simulink model "simscape_thermofluids_full"  (R2024b)
settings: Solver=VariableStepAuto  StartTime=0.0  StopTime=stopTime  FixedStep=timestep
values from neighbouring files (symbols this model uses):
  AC_tank_weight = AC_wall_thickness*AC_tank_surface_area*steel_density*2    [design_details.m]
  Ambient_temp = 300    [design_details.m]
  hose_length = 20    [design_details.m]
  Initial_temp = 300    [design_details.m]
  mass_per_length_supply = steel_density*wall_thickness*(supply_pipe_inner_area + supply_pipe_outer_area)    [design_details.m]
  supply_pipe_inner_diameter = 0.05    [design_details.m]
  wall_thickness = 2/1000    (= 0.002)    [design_details.m]
undefined symbols (not defined in the file or in its folder): AC_Bypass_SOV_POS, AC_Engine_SOV_POS, AC_Return_SOV_POS, AC_Supply_SOV_POS, GH2_PROP_VALVE_POS, GS_GH2_SOV_POS, GS_RETURN_PROP_POS, GS_Return_SOV_POS, GS_Supply_SOV_POS, LH2_PROP_VALVE_POS, mass_per_length_engine_feed, P_BYPASS, P_COUPLING_AC, P_COUPLING_AC_RETURN, P_COUPLINGS_GS, P_ENGINE_FEED, P_GH2_SUPPLY_GS, P_HOSE_GS, P_HOSE_RETURN_GS, P_PUMP_GS, P_SOV_RETURN_GS, P_TANK_AC, P_TANK_GS, P_VALVE_GS, T_BYPASS, T_COUPLING_AC, T_COUPLING_AC_RETURN, T_COUPLINGS_GS, T_ENGINE_FEED, T_GH2_SUPPLY_GS, T_HOSE_GS, T_HOSE_RETURN_GS, T_PUMP_GS, T_SOV_RETURN_GS, T_TANK_AC, T_TANK_GS, T_VALVE_GS
libraries: fl_lib x75, nesl_utility x62, SimscapeFluids_lib x14
(part 1 of 2)
settings Model: Creator=MW  LastModifiedBy=MW
settings SolverCC: SolverResetMethod=Robust

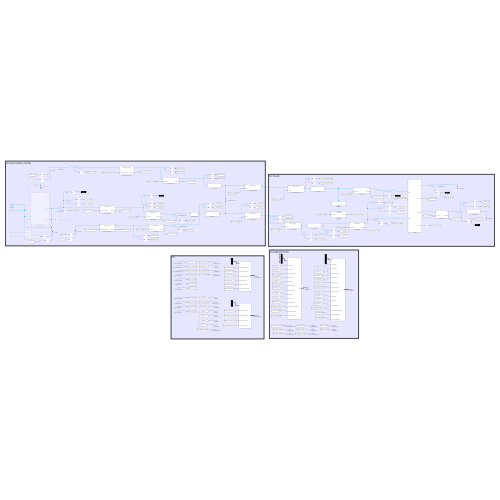
[thumbnail: Simulink's stored preview of the top-level diagram]
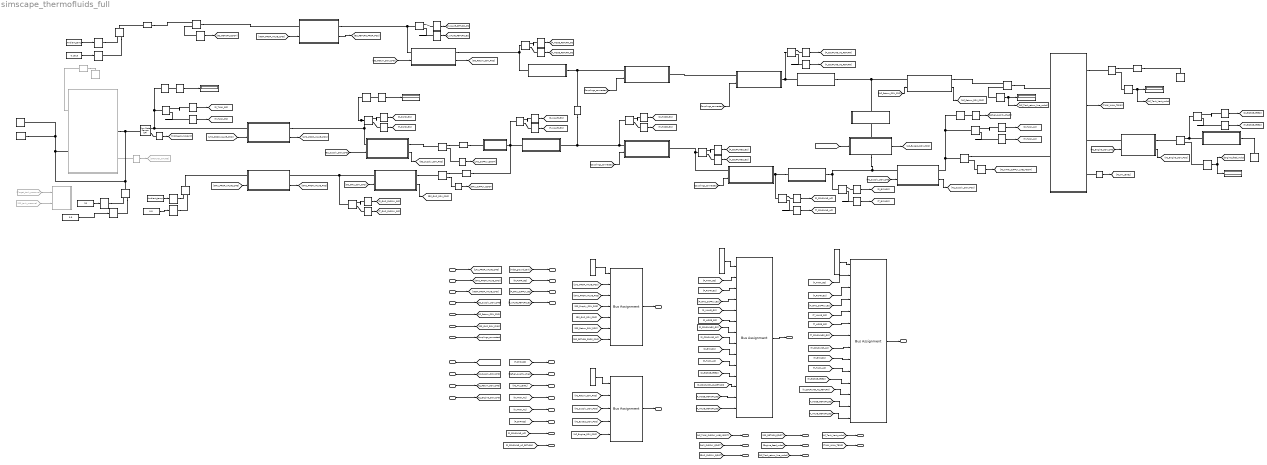
== system simscape_thermofluids_full ==
  note: Ground station fluids
  note: I/O
  note: AC fluids
  note: DIAGNOSTICS
  LH2_PROP_VALVE_CMD : Inport  OutDataTypeStr=double
  GH2_PROP_VALVE_CMD : Inport  Port=2
  VENT_PROP_VALVE_CMD : Inport  Port=3
  GS_Supply_SOV_CMD : Inport  Port=4  OutDataTypeStr=boolean
  GS_Return_SOV_CMD : Inport  Port=5  OutDataTypeStr=boolean
  GS_GH2_SOV_CMD : Inport  Port=6  OutDataTypeStr=boolean
  Couplings_connected : Inport  Port=7  OutDataTypeStr=boolean
  AC_Bypass_SOV_CMD : Inport  Port=8  OutDataTypeStr=boolean
  AC_Supply_SOV_CMD : Inport  Port=9  OutDataTypeStr=boolean
  AC_Return_SOV_CMD : Inport  Port=10  OutDataTypeStr=boolean
  AC_Engine_SOV_CMD : Inport  Port=11  OutDataTypeStr=boolean
  AC bypass check valve : SimscapeFluids_lib/Two-Phase Fluid/Valves & Orifices/Directional Control Valves/Check Valve (2P)  liquid_valve_parameterization=fluids.two_phase_fluid.valves_orifices.enum.LiquidPressureValveParameterization.LinearArea  opening_pressure_spec=fluids.two_phase_fluid.valves_orifices.enum.PressureControlSpec.PressureDifferential  p_crack_differential=1 bar  p_crack_gauge=0.1 MPa  p_max_differential=1.2 bar  p_max_gauge=0.2 MPa  mdot_nominal_max=0.1 kg/s  delta_p_nominal_max=0.001 MPa  valve_area_max=return_valve_orifice_area m^2  p_diff_TLU=[0.2 : 0.2 : 1.2] MPa  p_gauge_TLU=[0.2 : 0.2 : 1.2] MPa  valve_area_TLU=[1e-10, 2e-06, 4e-06, 6e-06, 8e-06, 1e-05] m^2  energy_spec=foundation.enum.energy_spec.temperature  p_inlet=0.101325 MPa  T_inlet=293.15 K  x_inlet=0  alpha_inlet=0  h_inlet=400 kJ/kg  u_inlet=400 kJ/kg  Cd=0.8  pressure_recovery=false  leakage_fraction=1e-9  smoothing_factor=0.01  B_lam=0.999  tau_x=0.1 s  area=return_pipe_inner_area m^2  vapor_valve_parameterization=fluids.two_phase_fluid.valves_orifices.enum.VaporOrificeParameterization.Cv  opening_characteristic=fluids.two_phase_fluid.valves_orifices.enum.OpeningCharacteristics.Linear  Cv_max=4  p_diff_Cv_TLU=0.2 : 0.2 : 1.2 MPa  p_gauge_Cv_TLU=0.2 : 0.2 : 1.2 MPa  Cv_TLU=[1e-06, .8, 1.6, 2.4, 3.2, 4]  xT_Cv=0.7  Kv_max=3.6  p_diff_Kv_TLU=0.2 : 0.2 : 1.2 MPa  p_gauge_Kv_TLU=0.2 : 0.2 : 1.2 MPa  Kv_TLU=[1e-06, .72, 1.44, 2.16, 2.88, 3.6]  xT_Kv=0.7  orifice_area_max=1e-4 m^2  p_diff_orifice_area_TLU=0.2 : 0.2 : 1.2 MPa  p_gauge_orifice_area_TLU=0.2 : 0.2 : 1.2 MPa  orifice_area_TLU=[1e-10, 2e-05, 4e-05, 6e-05, 8e-05, .0001] m^2
      settings: InternalSimscapePortConfiguration="{\"Bottom\":[],\"Left\":[{\"id\":\"A\",\"label\":\"A\",\"type\":\"foundation.two_phase_fluid.two_phase_fluid\"}],\"Right\":[{\"id\":\"B\",\"label\":\"B\",\"type\":\"foundation.two_phase_fluid.two_phase_fluid\"}],\"Top\":[]}"
  AC bypass pipe : Subsystem
      settings: PortSchema="{\"entries\":[{\"content\":{\"sides\":[{\"content\":{},\"type\":\"ConnectorPlacement.EquallySpacedRectSide\",\"uuid\":\"349fca2d-ac0c-44ed-9349-b644fbb08439\"},{\"content\":{\"side\":\"RIGHT\"},\"type\":\"ConnectorPlacement.EquallySpacedRectSide\",\"uuid\":\"6cc07318-8be0-4b72-ac83-45de534072f6\"},{\"content\":{\"connectorIds\":[\"LConn1\"],\"side\":\"TOP\"},\"type\":\"ConnectorPlacement.EquallySpacedRectSide\",\"uuid\":\"b4ae9877-c592-4d5d-8aa9-db7f627bda4a\"},{\"content\":{\"connectorIds\":[\"RConn1\"],\"side\":\"BOTTOM\"},\"type\":\"ConnectorPlacement.EquallySpacedRectSide\",\"uuid\":\"fa6d3200-a15a-4c5e-bc85-f306dce7b3ce\"}]},\"type\":\"ConnectorPlacement.EquallySpacedConnector\",\"uuid\":\"04c81fd1-333a-4337-ad58-fb71ace63568\"}],\"packageUris\":[\"http://schema.mathworks.com/mf0/Connector/R2020b\"],\"version\":\"1.0\"}"
  AC engine_feed_pipe : Subsystem
  AC return line pipe : Subsystem
  AC supply line pipe : Subsystem
  AC tank : Subsystem
      settings: PortSchema="{\"entries\":[{\"content\":{\"sides\":[{\"content\":{\"connectorIds\":[\"LConn1\",\"LConn2\"]},\"type\":\"ConnectorPlacement.EquallySpacedRectSide\",\"uuid\":\"18fbfd65-7892-4f33-871e-6daf68ba144c\"},{\"content\":{\"connectorIds\":[\"RConn1\",\"Out1\",\"RConn2\",\"RConn3\"],\"side\":\"RIGHT\"},\"type\":\"ConnectorPlacement.EquallySpacedRectSide\",\"uuid\":\"09c519c2-126c-4ac0-b88b-b8c0f8bd496e\"},{\"content\":{\"side\":\"TOP\"},\"type\":\"ConnectorPlacement.EquallySpacedRectSide\",\"uuid\":\"0da44e65-d94a-4bbc-a863-04d0cc4fadcc\"}]},\"type\":\"ConnectorPlacement.EquallySpacedConnector\",\"uuid\":\"f3f4eab3-fa1f-4341-9602-c44ab5467c31\"}],\"packageUris\":[\"http://schema.mathworks.com/mf0/Connector/R2020b\"],\"version\":\"1.0\"}"
  AC tank safety valve : SimscapeFluids_lib/Two-Phase Fluid/Valves & Orifices/Directional Control Valves/Check Valve (2P)  liquid_valve_parameterization=fluids.two_phase_fluid.valves_orifices.enum.LiquidPressureValveParameterization.LinearArea  opening_pressure_spec=fluids.two_phase_fluid.valves_orifices.enum.PressureControlSpec.PressureDifferential  p_crack_differential=5.5 bar  p_crack_gauge=0.1 MPa  p_max_differential=5.9 bar  p_max_gauge=0.2 MPa  mdot_nominal_max=0.1 kg/s  delta_p_nominal_max=0.001 MPa  valve_area_max=return_valve_orifice_area m^2  p_diff_TLU=[0.2 : 0.2 : 1.2] MPa  p_gauge_TLU=[0.2 : 0.2 : 1.2] MPa  valve_area_TLU=[1e-10, 2e-06, 4e-06, 6e-06, 8e-06, 1e-05] m^2  energy_spec=foundation.enum.energy_spec.temperature  p_inlet=0.101325 MPa  T_inlet=293.15 K  x_inlet=0  alpha_inlet=0  h_inlet=400 kJ/kg  u_inlet=400 kJ/kg  Cd=0.64  pressure_recovery=false  leakage_fraction=1e-9  smoothing_factor=0.01  B_lam=0.999  tau_x=0.1 s  area=return_pipe_inner_area m^2  vapor_valve_parameterization=fluids.two_phase_fluid.valves_orifices.enum.VaporOrificeParameterization.Cv  opening_characteristic=fluids.two_phase_fluid.valves_orifices.enum.OpeningCharacteristics.Linear  Cv_max=4  p_diff_Cv_TLU=0.2 : 0.2 : 1.2 MPa  p_gauge_Cv_TLU=0.2 : 0.2 : 1.2 MPa  Cv_TLU=[1e-06, .8, 1.6, 2.4, 3.2, 4]  xT_Cv=0.7  Kv_max=3.6  p_diff_Kv_TLU=0.2 : 0.2 : 1.2 MPa  p_gauge_Kv_TLU=0.2 : 0.2 : 1.2 MPa  Kv_TLU=[1e-06, .72, 1.44, 2.16, 2.88, 3.6]  xT_Kv=0.7  orifice_area_max=1e-4 m^2  p_diff_orifice_area_TLU=0.2 : 0.2 : 1.2 MPa  p_gauge_orifice_area_TLU=0.2 : 0.2 : 1.2 MPa  orifice_area_TLU=[1e-10, 2e-05, 4e-05, 6e-05, 8e-05, .0001] m^2
      settings: InternalSimscapePortConfiguration="{\"Bottom\":[],\"Left\":[{\"id\":\"A\",\"label\":\"A\",\"type\":\"foundation.two_phase_fluid.two_phase_fluid\"}],\"Right\":[{\"id\":\"B\",\"label\":\"B\",\"type\":\"foundation.two_phase_fluid.two_phase_fluid\"}],\"Top\":[]}"
  AC_Bypass_SOV : Subsystem  ReferencedSubsystem=liquid_supply_SOV
      settings: PortSchema="{\"entries\":[{\"content\":{\"sides\":[{\"content\":{\"connectorIds\":[\"In1\"]},\"type\":\"ConnectorPlacement.EquallySpacedRectSide\",\"uuid\":\"7761104f-7ea1-4b82-8256-1f0a81ecff04\"},{\"content\":{\"connectorIds\":[\"Out1\"],\"side\":\"RIGHT\"},\"type\":\"ConnectorPlacement.EquallySpacedRectSide\",\"uuid\":\"77ad54b1-fc7d-49b0-961f-dd624ba54eaa\"},{\"content\":{\"connectorIds\":[\"RConn1\"],\"side\":\"TOP\"},\"type\":\"ConnectorPlacement.EquallySpacedRectSide\",\"uuid\":\"3eb2c4da-9d99-4a14-9c12-4cb71cddfd05\"},{\"content\":{\"connectorIds\":[\"LConn1\"],\"side\":\"BOTTOM\"},\"type\":\"ConnectorPlacement.EquallySpacedRectSide\",\"uuid\":\"cc93d467-c3c5-4ce4-93ce-594b4fdbf767\"}]},\"type\":\"ConnectorPlacement.EquallySpacedConnector\",\"uuid\":\"a385487e-9e14-4b1e-bbba-76ef306222d1\"}],\"packageUris\":[\"http://schema.mathworks.com/mf0/Connector/R2020b\"],\"version\":\"1.0\"}"
  AC_Engine_SOV : Subsystem
      settings: PortSchema="{\"entries\":[{\"content\":{\"sides\":[{\"content\":{\"connectorIds\":[\"LConn1\",\"In1\"]},\"type\":\"ConnectorPlacement.EquallySpacedRectSide\",\"uuid\":\"8de00a24-9637-44f9-b77e-5b0008e83c26\"},{\"content\":{\"connectorIds\":[\"RConn1\",\"Out1\"],\"side\":\"RIGHT\"},\"type\":\"ConnectorPlacement.EquallySpacedRectSide\",\"uuid\":\"a538d446-b2a2-4ee6-8065-c38203dba177\"},{\"content\":{\"side\":\"TOP\"},\"type\":\"ConnectorPlacement.EquallySpacedRectSide\",\"uuid\":\"7c3a0b8e-131f-419e-9dd3-9151f58d9c4d\"}]},\"type\":\"ConnectorPlacement.EquallySpacedConnector\",\"uuid\":\"82546791-8f2d-494c-94b0-dfe79e322a77\"}],\"packageUris\":[\"http://schema.mathworks.com/mf0/Connector/R2020b\"],\"version\":\"1.0\"}"
  AC_Return_Coupling : Subsystem  ReferencedSubsystem=Return_coupling
      settings: PortSchema="{\"entries\":[{\"content\":{\"sides\":[{\"content\":{\"connectorIds\":[\"LConn1\",\"In1\"]},\"type\":\"ConnectorPlacement.EquallySpacedRectSide\",\"uuid\":\"1377ff57-d661-4db4-88bf-068b5be5647d\"},{\"content\":{\"connectorIds\":[\"RConn1\"],\"side\":\"RIGHT\"},\"type\":\"ConnectorPlacement.EquallySpacedRectSide\",\"uuid\":\"b2bd98a1-a4a4-4b83-ae68-33d4546d1bd4\"},{\"content\":{\"side\":\"TOP\"},\"type\":\"ConnectorPlacement.EquallySpacedRectSide\",\"uuid\":\"bd2d13e7-0124-4459-acb6-2626b7f191a3\"}]},\"type\":\"ConnectorPlacement.EquallySpacedConnector\",\"uuid\":\"1a0dd594-d6c0-4a46-87d8-aae9dae4eba9\"}],\"packageUris\":[\"http://schema.mathworks.com/mf0/Connector/R2020b\"],\"version\":\"1.0\"}"
  AC_Return_SOV : Subsystem
      settings: PortSchema="{\"entries\":[{\"content\":{\"sides\":[{\"content\":{\"connectorIds\":[\"LConn1\",\"In1\"]},\"type\":\"ConnectorPlacement.EquallySpacedRectSide\",\"uuid\":\"1377ff57-d661-4db4-88bf-068b5be5647d\"},{\"content\":{\"connectorIds\":[\"RConn1\",\"Out1\"],\"side\":\"RIGHT\"},\"type\":\"ConnectorPlacement.EquallySpacedRectSide\",\"uuid\":\"b2bd98a1-a4a4-4b83-ae68-33d4546d1bd4\"},{\"content\":{\"side\":\"TOP\"},\"type\":\"ConnectorPlacement.EquallySpacedRectSide\",\"uuid\":\"bd2d13e7-0124-4459-acb6-2626b7f191a3\"},{\"content\":{\"side\":\"BOTTOM\"},\"type\":\"ConnectorPlacement.EquallySpacedRectSide\",\"uuid\":\"65261db1-7dc3-4c3c-a5c1-ee0ef291cfbc\"}]},\"type\":\"ConnectorPlacement.EquallySpacedConnector\",\"uuid\":\"1a0dd594-d6c0-4a46-87d8-aae9dae4eba9\"}],\"packageUris\":[\"http://schema.mathworks.com/mf0/Connector/R2020b\"],\"version\":\"1.0\"}"
  AC_Supply_Coupling : Subsystem  ReferencedSubsystem=Supply_coupling
      settings: PortSchema="{\"entries\":[{\"content\":{\"sides\":[{\"content\":{\"connectorIds\":[\"LConn1\",\"In1\"]},\"type\":\"ConnectorPlacement.EquallySpacedRectSide\",\"uuid\":\"1377ff57-d661-4db4-88bf-068b5be5647d\"},{\"content\":{\"connectorIds\":[\"RConn1\"],\"side\":\"RIGHT\"},\"type\":\"ConnectorPlacement.EquallySpacedRectSide\",\"uuid\":\"b2bd98a1-a4a4-4b83-ae68-33d4546d1bd4\"},{\"content\":{\"side\":\"TOP\"},\"type\":\"ConnectorPlacement.EquallySpacedRectSide\",\"uuid\":\"bd2d13e7-0124-4459-acb6-2626b7f191a3\"}]},\"type\":\"ConnectorPlacement.EquallySpacedConnector\",\"uuid\":\"1a0dd594-d6c0-4a46-87d8-aae9dae4eba9\"}],\"packageUris\":[\"http://schema.mathworks.com/mf0/Connector/R2020b\"],\"version\":\"1.0\"}"
  AC_Supply_SOV : Subsystem  ReferencedSubsystem=liquid_supply_SOV
      settings: PortSchema="{\"entries\":[{\"content\":{\"sides\":[{\"content\":{\"connectorIds\":[\"LConn1\",\"In1\"]},\"type\":\"ConnectorPlacement.EquallySpacedRectSide\",\"uuid\":\"7761104f-7ea1-4b82-8256-1f0a81ecff04\"},{\"content\":{\"connectorIds\":[\"RConn1\",\"Out1\"],\"side\":\"RIGHT\"},\"type\":\"ConnectorPlacement.EquallySpacedRectSide\",\"uuid\":\"77ad54b1-fc7d-49b0-961f-dd624ba54eaa\"},{\"content\":{\"side\":\"TOP\"},\"type\":\"ConnectorPlacement.EquallySpacedRectSide\",\"uuid\":\"3eb2c4da-9d99-4a14-9c12-4cb71cddfd05\"}]},\"type\":\"ConnectorPlacement.EquallySpacedConnector\",\"uuid\":\"a385487e-9e14-4b1e-bbba-76ef306222d1\"}],\"packageUris\":[\"http://schema.mathworks.com/mf0/Connector/R2020b\"],\"version\":\"1.0\"}"
  Atmosphere : fl_lib/Two-Phase Fluid/Elements/Reservoir (2P)  Commented=on  pressure_spec=foundation.enum.ReservoirPressureSpec2P.Specified  reservoir_pressure=0.101325 MPa  reservoir_condensing_temperature=373.15 K  reservoir_evaporating_temperature=373.15 K  energy_spec=foundation.enum.ReservoirEnergySpec2P.Temperature  reservoir_temperature=Ambient_temp K  reservoir_quality=0.5  reservoir_void_fraction=0.5  reservoir_enthalpy=1500 kJ/kg  reservoir_internal_energy=1500 kJ/kg  reservoir_subcooling=5 deltaK  reservoir_superheating=5 deltaK  area_A=0.01 m^2
  Atmosphere2 : fl_lib/Two-Phase Fluid/Elements/Reservoir (2P)  pressure_spec=foundation.enum.ReservoirPressureSpec2P.Specified  reservoir_pressure=0.101325 MPa  reservoir_condensing_temperature=373.15 K  reservoir_evaporating_temperature=373.15 K  energy_spec=foundation.enum.ReservoirEnergySpec2P.Temperature  reservoir_temperature=293.15 K  reservoir_quality=0.5  reservoir_void_fraction=0.5  reservoir_enthalpy=1500 kJ/kg  reservoir_internal_energy=1500 kJ/kg  reservoir_subcooling=5 deltaK  reservoir_superheating=5 deltaK  area_A=0.02 m^2
  Atmosphere3 : fl_lib/Two-Phase Fluid/Elements/Reservoir (2P)  pressure_spec=foundation.enum.ReservoirPressureSpec2P.Specified  reservoir_pressure=0.101325 MPa  reservoir_condensing_temperature=373.15 K  reservoir_evaporating_temperature=373.15 K  energy_spec=foundation.enum.ReservoirEnergySpec2P.Temperature  reservoir_temperature=Ambient_temp K  reservoir_quality=0.5  reservoir_void_fraction=0.5  reservoir_enthalpy=1500 kJ/kg  reservoir_internal_energy=1500 kJ/kg  reservoir_subcooling=5 deltaK  reservoir_superheating=5 deltaK  area_A=engine_feed_pipe_inner_area m^2
  Bus Assignment : BusAssignment  AssignedSignals=P_TANK_GS,P_PUMP_GS,P_GH2_SUPPLY_GS,P_VALVE_GS,P_HOSE_GS,P_COUPLINGS_GS,P_COUPLING_AC,P_BYPASS,P_TANK_AC,P_ENGINE_FEED,P_COUPLING_AC_RETURN,P_HOSE_RETURN_GS,P_SOV_RETURN_GS
  Bus Assignment1 : BusAssignment  AssignedSignals=T_TANK_GS,T_PUMP_GS,T_GH2_SUPPLY_GS,T_VALVE_GS,T_HOSE_GS,T_COUPLINGS_GS,T_COUPLING_AC,T_BYPASS,T_TANK_AC,T_ENGINE_FEED,T_COUPLING_AC_RETURN,T_HOSE_RETURN_GS,T_SOV_RETURN_GS
  Bus Assignment2 : BusAssignment  AssignedSignals=LH2_PROP_VALVE_POS,GH2_PROP_VALVE_POS,GS_Supply_SOV_POS,GS_GH2_SOV_POS,GS_Return_SOV_POS,GS_RETURN_PROP_POS
  Bus Assignment3 : BusAssignment  AssignedSignals=AC_Return_SOV_POS,AC_Supply_SOV_POS,AC_Bypass_SOV_POS,AC_Engine_SOV_POS
  Bus Creator : BusCreator  Inputs=13  OutDataTypeStr=Bus: P_DIAGNOSTIC  NonVirtualBus=on
      settings: InheritFromInputs=off
  Bus Creator1 : BusCreator  Inputs=13  OutDataTypeStr=Bus: T_DIAGNOSTIC  NonVirtualBus=on
      settings: InheritFromInputs=off
  Bus Creator2 : BusCreator  Inputs=6  OutDataTypeStr=Bus: GS_VALVE_FEEDBACK  NonVirtualBus=on
      settings: InheritFromInputs=off
  Bus Creator3 : BusCreator  Inputs=4  OutDataTypeStr=Bus: AC_VALVE_FEEDBACK  NonVirtualBus=on
      settings: InheritFromInputs=off
  Constant : Constant  Value=Ambient_temp
  Constant1 : Constant  Value=20
  Constant2 : Constant  Value=Ambient_temp
  Constant4 : Constant  Value=0.5
  Constant5 : Constant  Value=0.1013
  Constant6 : Constant  Value=0.5
  Display{,1..4} (5 alike) : Display
  Flow Rate Sensor (2P) : fl_lib/Two-Phase Fluid/Sensors/Flow Rate Sensor (2P)  mass_flow_measure=false  volumetric_flow_measure=true  energy_flow_measure=false
      settings: InternalSimscapePortConfiguration="{\"Bottom\":[],\"Left\":[{\"id\":\"A\",\"label\":\"A\",\"type\":\"foundation.two_phase_fluid.two_phase_fluid\"}],\"Right\":[{\"id\":\"B\",\"label\":\"B\",\"type\":\"foundation.two_phase_fluid.two_phase_fluid\"},{\"id\":\"V\",\"label\":\"V\",\"type\":\"output\"}],\"Top\":[]}"
  Flow Rate Sensor (2P)1 : fl_lib/Two-Phase Fluid/Sensors/Flow Rate Sensor (2P)  mass_flow_measure=false  volumetric_flow_measure=true  energy_flow_measure=false
      settings: InternalSimscapePortConfiguration="{\"Bottom\":[],\"Left\":[{\"id\":\"A\",\"label\":\"A\",\"type\":\"foundation.two_phase_fluid.two_phase_fluid\"}],\"Right\":[{\"id\":\"B\",\"label\":\"B\",\"type\":\"foundation.two_phase_fluid.two_phase_fluid\"},{\"id\":\"V\",\"label\":\"V\",\"type\":\"output\"}],\"Top\":[]}"
  Flow Rate Sensor (2P){2..3,5..6} (4 alike) : fl_lib/Two-Phase Fluid/Sensors/Flow Rate Sensor (2P)  mass_flow_measure=true  volumetric_flow_measure=false  energy_flow_measure=false
      settings: InternalSimscapePortConfiguration="{\"Bottom\":[],\"Left\":[{\"id\":\"A\",\"label\":\"A\",\"type\":\"foundation.two_phase_fluid.two_phase_fluid\"}],\"Right\":[{\"id\":\"B\",\"label\":\"B\",\"type\":\"foundation.two_phase_fluid.two_phase_fluid\"},{\"id\":\"M\",\"label\":\"M\",\"type\":\"output\"}],\"Top\":[]}"
  Flow Rate Sensor (2P)4 : fl_lib/Two-Phase Fluid/Sensors/Flow Rate Sensor (2P)  mass_flow_measure=false  volumetric_flow_measure=true  energy_flow_measure=false
      settings: InternalSimscapePortConfiguration="{\"Bottom\":[],\"Left\":[{\"id\":\"A\",\"label\":\"A\",\"type\":\"foundation.two_phase_fluid.two_phase_fluid\"}],\"Right\":[{\"id\":\"B\",\"label\":\"B\",\"type\":\"foundation.two_phase_fluid.two_phase_fluid\"},{\"id\":\"V\",\"label\":\"V\",\"type\":\"output\"}],\"Top\":[]}"
  Flow rate sensor : fl_lib/Two-Phase Fluid/Sensors/Flow Rate Sensor (2P)  mass_flow_measure=true  volumetric_flow_measure=false  energy_flow_measure=false
      settings: InternalSimscapePortConfiguration="{\"Bottom\":[],\"Left\":[{\"id\":\"A\",\"label\":\"A\",\"type\":\"foundation.two_phase_fluid.two_phase_fluid\"}],\"Right\":[{\"id\":\"B\",\"label\":\"B\",\"type\":\"foundation.two_phase_fluid.two_phase_fluid\"},{\"id\":\"M\",\"label\":\"M\",\"type\":\"output\"}],\"Top\":[]}"
  From : From  Commented=on  GotoTag=Target_tank_pressure
  From14 : From  Commented=on  GotoTag=GS_tank_pressure
  GH2 Proportional valve : Subsystem  ReferencedSubsystem=Gas_prop_valve
      settings: PortSchema="{\"entries\":[{\"content\":{\"sides\":[{\"content\":{\"connectorIds\":[\"LConn1\",\"In1\"]},\"type\":\"ConnectorPlacement.EquallySpacedRectSide\",\"uuid\":\"7761104f-7ea1-4b82-8256-1f0a81ecff04\"},{\"content\":{\"connectorIds\":[\"LConn2\",\"Out1\"],\"side\":\"RIGHT\"},\"type\":\"ConnectorPlacement.EquallySpacedRectSide\",\"uuid\":\"77ad54b1-fc7d-49b0-961f-dd624ba54eaa\"},{\"content\":{\"side\":\"TOP\"},\"type\":\"ConnectorPlacement.EquallySpacedRectSide\",\"uuid\":\"3eb2c4da-9d99-4a14-9c12-4cb71cddfd05\"},{\"content\":{\"side\":\"BOTTOM\"},\"type\":\"ConnectorPlacement.EquallySpacedRectSide\",\"uuid\":\"e49cc93b-8c4a-4262-8b13-a5abe2820965\"}]},\"type\":\"ConnectorPlacement.EquallySpacedConnector\",\"uuid\":\"a385487e-9e14-4b1e-bbba-76ef306222d1\"}],\"packageUris\":[\"http://schema.mathworks.com/mf0/Connector/R2020b\"],\"version\":\"1.0\"}"
  GH2 source : fl_lib/Two-Phase Fluid/Elements/Controlled Reservoir (2P)  pressure_spec=foundation.enum.ControlledReservoirPressureSpec2P.Specified  energy_spec=foundation.enum.ControlledReservoirEnergySpec2P.VaporTemperature  area_A=supply_valve_orifice_area m^2  pressure_limit_spec=foundation.enum.PressureLimitSpec2P.Warn
      settings: InternalSimscapePortConfiguration="{\"Bottom\":[],\"Left\":[{\"id\":\"A\",\"label\":\"A\",\"type\":\"foundation.two_phase_fluid.two_phase_fluid\"}],\"Right\":[{\"id\":\"T\",\"label\":\"T\",\"type\":\"input\"},{\"id\":\"P\",\"label\":\"P\",\"type\":\"input\"}],\"Top\":[]}"
  GH2 supply check valve : SimscapeFluids_lib/Two-Phase Fluid/Valves & Orifices/Directional Control Valves/Check Valve (2P)  liquid_valve_parameterization=fluids.two_phase_fluid.valves_orifices.enum.LiquidPressureValveParameterization.LinearArea  opening_pressure_spec=fluids.two_phase_fluid.valves_orifices.enum.PressureControlSpec.PressureDifferential  p_crack_differential=0.01 bar  p_crack_gauge=0.1 MPa  p_max_differential=0.03 bar  p_max_gauge=0.2 MPa  mdot_nominal_max=0.1 kg/s  delta_p_nominal_max=0.001 MPa  valve_area_max=supply_valve_orifice_area m^2  p_diff_TLU=[0.2 : 0.2 : 1.2] MPa  p_gauge_TLU=[0.2 : 0.2 : 1.2] MPa  valve_area_TLU=[1e-10, 2e-06, 4e-06, 6e-06, 8e-06, 1e-05] m^2  energy_spec=foundation.enum.energy_spec.temperature  p_inlet=0.101325 MPa  T_inlet=293.15 K  x_inlet=0  alpha_inlet=0  h_inlet=400 kJ/kg  u_inlet=400 kJ/kg  Cd=0.8  pressure_recovery=false  leakage_fraction=1e-9  smoothing_factor=0.01  B_lam=0.999  tau_x=0.1 s  area=supply_pipe_inner_area m^2  vapor_valve_parameterization=fluids.two_phase_fluid.valves_orifices.enum.VaporOrificeParameterization.Cv  opening_characteristic=fluids.two_phase_fluid.valves_orifices.enum.OpeningCharacteristics.Linear  Cv_max=4  p_diff_Cv_TLU=0.2 : 0.2 : 1.2 MPa  p_gauge_Cv_TLU=0.2 : 0.2 : 1.2 MPa  Cv_TLU=[1e-06, .8, 1.6, 2.4, 3.2, 4]  xT_Cv=0.7  Kv_max=3.6  p_diff_Kv_TLU=0.2 : 0.2 : 1.2 MPa  p_gauge_Kv_TLU=0.2 : 0.2 : 1.2 MPa  Kv_TLU=[1e-06, .72, 1.44, 2.16, 2.88, 3.6]  xT_Kv=0.7  orifice_area_max=1e-4 m^2  p_diff_orifice_area_TLU=0.2 : 0.2 : 1.2 MPa  p_gauge_orifice_area_TLU=0.2 : 0.2 : 1.2 MPa  orifice_area_TLU=[1e-10, 2e-05, 4e-05, 6e-05, 8e-05, .0001] m^2
      settings: InternalSimscapePortConfiguration="{\"Bottom\":[],\"Left\":[{\"id\":\"A\",\"label\":\"A\",\"type\":\"foundation.two_phase_fluid.two_phase_fluid\"}],\"Right\":[{\"id\":\"B\",\"label\":\"B\",\"type\":\"foundation.two_phase_fluid.two_phase_fluid\"}],\"Top\":[]}"
  GH2 vent : fl_lib/Two-Phase Fluid/Elements/Controlled Reservoir (2P)  pressure_spec=foundation.enum.ControlledReservoirPressureSpec2P.Specified  energy_spec=foundation.enum.ControlledReservoirEnergySpec2P.VaporTemperature  area_A=supply_valve_orifice_area m^2  pressure_limit_spec=foundation.enum.PressureLimitSpec2P.Warn
      settings: InternalSimscapePortConfiguration="{\"Bottom\":[],\"Left\":[{\"id\":\"A\",\"label\":\"A\",\"type\":\"foundation.two_phase_fluid.two_phase_fluid\"}],\"Right\":[{\"id\":\"T\",\"label\":\"T\",\"type\":\"input\"},{\"id\":\"P\",\"label\":\"P\",\"type\":\"input\"}],\"Top\":[]}"
  GS supply line pipe : Subsystem
  GS tank pressure controller : Subsystem  Commented=on
  GS_GH2_SOV : Subsystem  ReferencedSubsystem=liquid_supply_SOV
      settings: PortSchema="{\"entries\":[{\"content\":{\"sides\":[{\"content\":{\"connectorIds\":[\"LConn1\",\"In1\"]},\"type\":\"ConnectorPlacement.EquallySpacedRectSide\",\"uuid\":\"7761104f-7ea1-4b82-8256-1f0a81ecff04\"},{\"content\":{\"connectorIds\":[\"RConn1\",\"Out1\"],\"side\":\"RIGHT\"},\"type\":\"ConnectorPlacement.EquallySpacedRectSide\",\"uuid\":\"77ad54b1-fc7d-49b0-961f-dd624ba54eaa\"},{\"content\":{\"side\":\"TOP\"},\"type\":\"ConnectorPlacement.EquallySpacedRectSide\",\"uuid\":\"3eb2c4da-9d99-4a14-9c12-4cb71cddfd05\"}]},\"type\":\"ConnectorPlacement.EquallySpacedConnector\",\"uuid\":\"a385487e-9e14-4b1e-bbba-76ef306222d1\"}],\"packageUris\":[\"http://schema.mathworks.com/mf0/Connector/R2020b\"],\"version\":\"1.0\"}"
  GS_Return_Coupling : Subsystem  ReferencedSubsystem=Return_coupling
      settings: PortSchema="{\"entries\":[{\"content\":{\"sides\":[{\"content\":{\"connectorIds\":[\"LConn1\",\"In1\"]},\"type\":\"ConnectorPlacement.EquallySpacedRectSide\",\"uuid\":\"1377ff57-d661-4db4-88bf-068b5be5647d\"},{\"content\":{\"connectorIds\":[\"RConn1\"],\"side\":\"RIGHT\"},\"type\":\"ConnectorPlacement.EquallySpacedRectSide\",\"uuid\":\"b2bd98a1-a4a4-4b83-ae68-33d4546d1bd4\"},{\"content\":{\"side\":\"TOP\"},\"type\":\"ConnectorPlacement.EquallySpacedRectSide\",\"uuid\":\"bd2d13e7-0124-4459-acb6-2626b7f191a3\"}]},\"type\":\"ConnectorPlacement.EquallySpacedConnector\",\"uuid\":\"1a0dd594-d6c0-4a46-87d8-aae9dae4eba9\"}],\"packageUris\":[\"http://schema.mathworks.com/mf0/Connector/R2020b\"],\"version\":\"1.0\"}"
  GS_Return_SOV : Subsystem
      settings: PortSchema="{\"entries\":[{\"content\":{\"sides\":[{\"content\":{\"connectorIds\":[\"LConn1\",\"In1\"]},\"type\":\"ConnectorPlacement.EquallySpacedRectSide\",\"uuid\":\"1377ff57-d661-4db4-88bf-068b5be5647d\"},{\"content\":{\"connectorIds\":[\"RConn1\",\"Out1\"],\"side\":\"RIGHT\"},\"type\":\"ConnectorPlacement.EquallySpacedRectSide\",\"uuid\":\"b2bd98a1-a4a4-4b83-ae68-33d4546d1bd4\"},{\"content\":{\"side\":\"TOP\"},\"type\":\"ConnectorPlacement.EquallySpacedRectSide\",\"uuid\":\"bd2d13e7-0124-4459-acb6-2626b7f191a3\"}]},\"type\":\"ConnectorPlacement.EquallySpacedConnector\",\"uuid\":\"1a0dd594-d6c0-4a46-87d8-aae9dae4eba9\"}],\"packageUris\":[\"http://schema.mathworks.com/mf0/Connector/R2020b\"],\"version\":\"1.0\"}"
  GS_Supply_Coupling : Subsystem  ReferencedSubsystem=Supply_coupling
      settings: PortSchema="{\"entries\":[{\"content\":{\"sides\":[{\"content\":{\"connectorIds\":[\"LConn1\",\"In1\"]},\"type\":\"ConnectorPlacement.EquallySpacedRectSide\",\"uuid\":\"1377ff57-d661-4db4-88bf-068b5be5647d\"},{\"content\":{\"connectorIds\":[\"RConn1\"],\"side\":\"RIGHT\"},\"type\":\"ConnectorPlacement.EquallySpacedRectSide\",\"uuid\":\"b2bd98a1-a4a4-4b83-ae68-33d4546d1bd4\"},{\"content\":{\"side\":\"TOP\"},\"type\":\"ConnectorPlacement.EquallySpacedRectSide\",\"uuid\":\"bd2d13e7-0124-4459-acb6-2626b7f191a3\"}]},\"type\":\"ConnectorPlacement.EquallySpacedConnector\",\"uuid\":\"1a0dd594-d6c0-4a46-87d8-aae9dae4eba9\"}],\"packageUris\":[\"http://schema.mathworks.com/mf0/Connector/R2020b\"],\"version\":\"1.0\"}"
  GS_Supply_SOV : Subsystem  ReferencedSubsystem=liquid_supply_SOV
      settings: PortSchema="{\"entries\":[{\"content\":{\"sides\":[{\"content\":{\"connectorIds\":[\"LConn1\",\"In1\"]},\"type\":\"ConnectorPlacement.EquallySpacedRectSide\",\"uuid\":\"7761104f-7ea1-4b82-8256-1f0a81ecff04\"},{\"content\":{\"connectorIds\":[\"RConn1\",\"Out1\"],\"side\":\"RIGHT\"},\"type\":\"ConnectorPlacement.EquallySpacedRectSide\",\"uuid\":\"77ad54b1-fc7d-49b0-961f-dd624ba54eaa\"},{\"content\":{\"side\":\"TOP\"},\"type\":\"ConnectorPlacement.EquallySpacedRectSide\",\"uuid\":\"3eb2c4da-9d99-4a14-9c12-4cb71cddfd05\"}]},\"type\":\"ConnectorPlacement.EquallySpacedConnector\",\"uuid\":\"a385487e-9e14-4b1e-bbba-76ef306222d1\"}],\"packageUris\":[\"http://schema.mathworks.com/mf0/Connector/R2020b\"],\"version\":\"1.0\"}"
  Goto1 : Goto  Commented=on  GotoTag=GROUND_GAUGE
  Ground station tank : Subsystem  Commented=on
  H2 2 phase : fl_lib/Two-Phase Fluid/Utilities/Two-Phase Fluid Properties (2P)  u_min=H2Tables.u_min kJ/kg  u_max=H2Tables.u_max kJ/kg  p_TLU=H2Tables.p MPa  p_crit=H2Tables.p_crit MPa  critical_region=foundation.enum.critical_region.clip  p_crit_fraction=0.12  p_atm=0.101325 MPa  properties_range_check=simscape.enum.assert.action.error  q_rev=0.01 Pa  unorm_liq=H2Tables.liquid.unorm  v_liq=H2Tables.liquid.v m^3/kg  s_liq=H2Tables.liquid.s kJ/(kg*K)  T_liq=H2Tables.liquid.T K  nu_liq=H2Tables.liquid.nu mm^2/s  k_liq=H2Tables.liquid.k W/(m*K)  Pr_liq=H2Tables.liquid.Pr  u_sat_liq=H2Tables.liquid.u_sat kJ/kg  unorm_vap=H2Tables.vapor.unorm  v_vap=H2Tables.vapor.v m^3/kg  s_vap=H2Tables.vapor.s kJ/(kg*K)  T_vap=H2Tables.vapor.T K  nu_vap=H2Tables.vapor.nu mm^2/s  k_vap=H2Tables.vapor.k W/(m*K)  Pr_vap=H2Tables.vapor.Pr  u_sat_vap=H2Tables.vapor.u_sat kJ/kg
      settings: InternalSimscapePortConfiguration="{\"Bottom\":[],\"Left\":[],\"Right\":[{\"id\":\"A\",\"label\":\"\",\"type\":\"foundation.two_phase_fluid.two_phase_fluid\"}],\"Top\":[]}"
  LH2 Proportional valve : Subsystem  ReferencedSubsystem=LH2_prop_valve
      settings: PortSchema="{\"entries\":[{\"content\":{\"sides\":[{\"content\":{\"connectorIds\":[\"LConn1\",\"In1\"]},\"type\":\"ConnectorPlacement.EquallySpacedRectSide\",\"uuid\":\"feebead4-63a3-41be-b6af-c9093fc48b74\"},{\"content\":{\"connectorIds\":[\"LConn2\",\"Out1\"],\"side\":\"RIGHT\"},\"type\":\"ConnectorPlacement.EquallySpacedRectSide\",\"uuid\":\"7fa0aa45-6202-479f-80c3-49b7dbf56766\"},{\"content\":{\"side\":\"TOP\"},\"type\":\"ConnectorPlacement.EquallySpacedRectSide\",\"uuid\":\"fffd3c2c-2b50-47ce-80c6-79193e21f29e\"},{\"content\":{\"side\":\"BOTTOM\"},\"type\":\"ConnectorPlacement.EquallySpacedRectSide\",\"uuid\":\"957ddecd-60b1-4a90-a8a1-75fcc228f543\"}]},\"type\":\"ConnectorPlacement.EquallySpacedConnector\",\"uuid\":\"476b1e20-77c8-4bf2-b4c4-536305065543\"}],\"packageUris\":[\"http://schema.mathworks.com/mf0/Connector/R2020b\"],\"version\":\"1.0\"}"
  LH2 source : fl_lib/Two-Phase Fluid/Elements/Controlled Reservoir (2P)  pressure_spec=foundation.enum.ControlledReservoirPressureSpec2P.Specified  energy_spec=foundation.enum.ControlledReservoirEnergySpec2P.LiquidTemperature  area_A=0.1 m^2  pressure_limit_spec=foundation.enum.PressureLimitSpec2P.Limit
      settings: InternalSimscapePortConfiguration="{\"Bottom\":[],\"Left\":[{\"id\":\"A\",\"label\":\"A\",\"type\":\"foundation.two_phase_fluid.two_phase_fluid\"}],\"Right\":[{\"id\":\"T\",\"label\":\"T\",\"type\":\"input\"},{\"id\":\"P\",\"label\":\"P\",\"type\":\"input\"}],\"Top\":[]}"
  LH2 supply check valve : SimscapeFluids_lib/Two-Phase Fluid/Valves & Orifices/Directional Control Valves/Check Valve (2P)  liquid_valve_parameterization=fluids.two_phase_fluid.valves_orifices.enum.LiquidPressureValveParameterization.LinearArea  opening_pressure_spec=fluids.two_phase_fluid.valves_orifices.enum.PressureControlSpec.PressureDifferential  p_crack_differential=0.01 bar  p_crack_gauge=0.1 MPa  p_max_differential=0.03 bar  p_max_gauge=0.2 MPa  mdot_nominal_max=0.1 kg/s  delta_p_nominal_max=0.001 MPa  valve_area_max=supply_valve_orifice_area m^2  p_diff_TLU=[0.2 : 0.2 : 1.2] MPa  p_gauge_TLU=[0.2 : 0.2 : 1.2] MPa  valve_area_TLU=[1e-10, 2e-06, 4e-06, 6e-06, 8e-06, 1e-05] m^2  energy_spec=foundation.enum.energy_spec.temperature  p_inlet=0.101325 MPa  T_inlet=293.15 K  x_inlet=0  alpha_inlet=0  h_inlet=400 kJ/kg  u_inlet=400 kJ/kg  Cd=0.8  pressure_recovery=false  leakage_fraction=1e-9  smoothing_factor=0.01  B_lam=0.999  tau_x=0.1 s  area=supply_pipe_inner_area m^2  vapor_valve_parameterization=fluids.two_phase_fluid.valves_orifices.enum.VaporOrificeParameterization.Cv  opening_characteristic=fluids.two_phase_fluid.valves_orifices.enum.OpeningCharacteristics.Linear  Cv_max=4  p_diff_Cv_TLU=0.2 : 0.2 : 1.2 MPa  p_gauge_Cv_TLU=0.2 : 0.2 : 1.2 MPa  Cv_TLU=[1e-06, .8, 1.6, 2.4, 3.2, 4]  xT_Cv=0.7  Kv_max=3.6  p_diff_Kv_TLU=0.2 : 0.2 : 1.2 MPa  p_gauge_Kv_TLU=0.2 : 0.2 : 1.2 MPa  Kv_TLU=[1e-06, .72, 1.44, 2.16, 2.88, 3.6]  xT_Kv=0.7  orifice_area_max=1e-4 m^2  p_diff_orifice_area_TLU=0.2 : 0.2 : 1.2 MPa  p_gauge_orifice_area_TLU=0.2 : 0.2 : 1.2 MPa  orifice_area_TLU=[1e-10, 2e-05, 4e-05, 6e-05, 8e-05, .0001] m^2
      settings: InternalSimscapePortConfiguration="{\"Bottom\":[],\"Left\":[{\"id\":\"A\",\"label\":\"A\",\"type\":\"foundation.two_phase_fluid.two_phase_fluid\"}],\"Right\":[{\"id\":\"B\",\"label\":\"B\",\"type\":\"foundation.two_phase_fluid.two_phase_fluid\"}],\"Top\":[]}"
  PS-Simulink Converter{,1,3..38} (38 alike) : nesl_utility/PS-Simulink Converter  PhysicalDomain=network_engine_domain  SubClassName=ps_output  LeftPortType=input  RightPortType=output  PseudoPeriodic=off  Frequencies=[]  VectorFormat=inherit  Unit=inherit  AffineConversion=off
  PS-Simulink Converter2 : nesl_utility/PS-Simulink Converter  Commented=on  PhysicalDomain=network_engine_domain  SubClassName=ps_output  LeftPortType=input  RightPortType=output  PseudoPeriodic=off  Frequencies=[]  VectorFormat=inherit  Unit=inherit  AffineConversion=off
  Pressure, Temperature & Internal Energy Sensor (2P){,1..12} (13 alike) : fl_lib/Two-Phase Fluid/Sensors/Pressure, Temperature & Internal Energy Sensor (2P)  reference=foundation.enum.MeasurementReference.absolute  pressure=true  pressure_spec=foundation.enum.PressureMeasementSpec.Absolute  temperature=true  internal_energy=false
      settings: InternalSimscapePortConfiguration="{\"Bottom\":[{\"id\":\"T\",\"label\":\"T\",\"type\":\"output\"}],\"Left\":[{\"id\":\"A\",\"label\":\"A\",\"type\":\"foundation.two_phase_fluid.two_phase_fluid\"}],\"Right\":[{\"id\":\"Pa\",\"label\":\"Pa\",\"type\":\"output\"}],\"Top\":[]}"
  Return gas proportional valve : Subsystem  ReferencedSubsystem=Return_gas_prop_valve
      settings: PortSchema="{\"entries\":[{\"content\":{\"sides\":[{\"content\":{\"connectorIds\":[\"LConn2\",\"In1\"]},\"type\":\"ConnectorPlacement.EquallySpacedRectSide\",\"uuid\":\"7b60590b-4a7b-465d-b616-9ce36d4c9bd1\"},{\"content\":{\"connectorIds\":[\"LConn1\",\"Out1\"],\"side\":\"RIGHT\"},\"type\":\"ConnectorPlacement.EquallySpacedRectSide\",\"uuid\":\"021f4d26-2a2b-40fc-b211-2c38ffe0620d\"},{\"content\":{\"side\":\"TOP\"},\"type\":\"ConnectorPlacement.EquallySpacedRectSide\",\"uuid\":\"273f71b8-2e8c-4f2f-b50f-0419d15b1792\"}]},\"type\":\"ConnectorPlacement.EquallySpacedConnector\",\"uuid\":\"b42a82ba-0baa-43b5-8ff8-ec1372f42070\"}],\"packageUris\":[\"http://schema.mathworks.com/mf0/Connector/R2020b\"],\"version\":\"1.0\"}"
  Return line hose : Subsystem
  Safety valve : SimscapeFluids_lib/Two-Phase Fluid/Valves & Orifices/Directional Control Valves/Check Valve (2P)  Commented=on  liquid_valve_parameterization=fluids.two_phase_fluid.valves_orifices.enum.LiquidPressureValveParameterization.LinearArea  opening_pressure_spec=fluids.two_phase_fluid.valves_orifices.enum.PressureControlSpec.PressureDifferential  p_crack_differential=6 bar  p_crack_gauge=0.1 MPa  p_max_differential=7 bar  p_max_gauge=0.2 MPa  mdot_nominal_max=0.1 kg/s  delta_p_nominal_max=0.001 MPa  valve_area_max=1e-2 m^2  p_diff_TLU=[0.2 : 0.2 : 1.2] MPa  p_gauge_TLU=[0.2 : 0.2 : 1.2] MPa  valve_area_TLU=[1e-10, 2e-06, 4e-06, 6e-06, 8e-06, 1e-05] m^2  energy_spec=foundation.enum.energy_spec.temperature  p_inlet=0.101325 MPa  T_inlet=293.15 K  x_inlet=0  alpha_inlet=0  h_inlet=400 kJ/kg  u_inlet=400 kJ/kg  Cd=0.64  pressure_recovery=false  leakage_fraction=1e-9  smoothing_factor=0.01  B_lam=0.999  tau_x=0.1 s  area=0.02 m^2  vapor_valve_parameterization=fluids.two_phase_fluid.valves_orifices.enum.VaporOrificeParameterization.Cv  opening_characteristic=fluids.two_phase_fluid.valves_orifices.enum.OpeningCharacteristics.Linear  Cv_max=4  p_diff_Cv_TLU=0.2 : 0.2 : 1.2 MPa  p_gauge_Cv_TLU=0.2 : 0.2 : 1.2 MPa  Cv_TLU=[1e-06, .8, 1.6, 2.4, 3.2, 4]  xT_Cv=0.7  Kv_max=3.6  p_diff_Kv_TLU=0.2 : 0.2 : 1.2 MPa  p_gauge_Kv_TLU=0.2 : 0.2 : 1.2 MPa  Kv_TLU=[1e-06, .72, 1.44, 2.16, 2.88, 3.6]  xT_Kv=0.7  orifice_area_max=1e-4 m^2  p_diff_orifice_area_TLU=0.2 : 0.2 : 1.2 MPa  p_gauge_orifice_area_TLU=0.2 : 0.2 : 1.2 MPa  orifice_area_TLU=[1e-10, 2e-05, 4e-05, 6e-05, 8e-05, .0001] m^2
      settings: InternalSimscapePortConfiguration="{\"Bottom\":[],\"Left\":[{\"id\":\"A\",\"label\":\"A\",\"type\":\"foundation.two_phase_fluid.two_phase_fluid\"}],\"Right\":[{\"id\":\"B\",\"label\":\"B\",\"type\":\"foundation.two_phase_fluid.two_phase_fluid\"}],\"Top\":[]}"
  Simulink-PS Converter{,1..5} (6 alike) : nesl_utility/Simulink-PS Converter  PhysicalDomain=network_engine_domain  SubClassName=ps_input  LeftPortType=input  RightPortType=output  PseudoPeriodic=off  Frequencies=[]  NoiseDistribution=none  NoiseParameters=[]  Unit=1  AffineConversion=off  FilteringAndDerivatives=provide  SimscapeFilterOrder=1  InputFilterTimeConstant=0.001  UdotUserProvided=0
  Solver Configuration2 : nesl_utility/Solver Configuration  PhysicalDomain=network_engine_domain  SubClassName=solver  LeftPortType=input  RightPortType=generic  Tones=[]  Harmonics=[]  SimulateNoise=off  Profile=off  UseLocalSampling=off  EnableSwitchedLinearOptims=on  FrequencyDomain=off  UseCCode=off  RelTol=0.001  AbsTol=0.001  MinStep=1e-09  ToWorkspace=off  RevertToSquareIcSolve=off  NumHomotopyIterations=100  PhasorMode=off  PhasorModeNumHarmonics=1  ConsistencySolver=NEWTON_XTOL_AFTER_FTOL  IndexReductionMethod=DerivativeReplacement  DoDC=off  ResidualTolerance=1e-09  ConsistencyTolSource=GLOBAL  ConsistencyAbsTol=0.001  ConsistencyRelTol=0.001  ConsistencyTolFactor=1e-7  UseLocalSolver=off  LocalSolverChoice=NE_TRAPEZOIDAL_ADVANCER  ResolveIndetEquations=on  FunctionEvalNumThread=1  LocalSolverSampleTime=1e-3  DoFixedCost=off  MaxNonlinIter=3  MaxModeIter=2  ComputeImpulses=off  ImpulseIterations=2  LinearAlgebra=auto  LinearAlgebraNumThread=0  EquationFormulation=NE_TIME_EF  DelaysMemoryBudget=1024  AutomaticFiltering=on  FilteringTimeConstant=0.001  PartitionStorageMethod=AS_NEEDED  PartitionMemoryBudget=1024  PartitionMethod=ROBUST  MultibodyUseLocalSolver=off  MultibodyLocalSolverChoice=ODE1  MultibodyLocalSolverSampleTime=0.001
  Vapor Quality Sensor (2P) : fl_lib/Two-Phase Fluid/Sensors/Vapor Quality Sensor (2P)  vapor_fraction_spec=foundation.enum.vapor_fraction_spec.quality
      settings: InternalSimscapePortConfiguration="{\"Bottom\":[],\"Left\":[{\"id\":\"A\",\"label\":\"A\",\"type\":\"foundation.two_phase_fluid.two_phase_fluid\"}],\"Right\":[{\"id\":\"X\",\"label\":\"X\",\"type\":\"output\"}],\"Top\":[]}"
  Vapor Quality Sensor (2P)1 : fl_lib/Two-Phase Fluid/Sensors/Vapor Quality Sensor (2P)  vapor_fraction_spec=foundation.enum.vapor_fraction_spec.quality
      settings: InternalSimscapePortConfiguration="{\"Bottom\":[],\"Left\":[{\"id\":\"A\",\"label\":\"A\",\"type\":\"foundation.two_phase_fluid.two_phase_fluid\"}],\"Right\":[{\"id\":\"X\",\"label\":\"X\",\"type\":\"output\"}],\"Top\":[]}"
  Vapor Quality Sensor (2P)2 : fl_lib/Two-Phase Fluid/Sensors/Vapor Quality Sensor (2P)  vapor_fraction_spec=foundation.enum.vapor_fraction_spec.quality
      settings: InternalSimscapePortConfiguration="{\"Bottom\":[],\"Left\":[{\"id\":\"A\",\"label\":\"A\",\"type\":\"foundation.two_phase_fluid.two_phase_fluid\"}],\"Right\":[{\"id\":\"X\",\"label\":\"X\",\"type\":\"output\"}],\"Top\":[]}"
  Vent check valve : SimscapeFluids_lib/Two-Phase Fluid/Valves & Orifices/Directional Control Valves/Check Valve (2P)  liquid_valve_parameterization=fluids.two_phase_fluid.valves_orifices.enum.LiquidPressureValveParameterization.LinearArea  opening_pressure_spec=fluids.two_phase_fluid.valves_orifices.enum.PressureControlSpec.PressureDifferential  p_crack_differential=0.01 bar  p_crack_gauge=0.1 MPa  p_max_differential=0.03 bar  p_max_gauge=0.2 MPa  mdot_nominal_max=0.1 kg/s  delta_p_nominal_max=0.001 MPa  valve_area_max=return_valve_orifice_area m^2  p_diff_TLU=[0.2 : 0.2 : 1.2] MPa  p_gauge_TLU=[0.2 : 0.2 : 1.2] MPa  valve_area_TLU=[1e-10, 2e-06, 4e-06, 6e-06, 8e-06, 1e-05] m^2  energy_spec=foundation.enum.energy_spec.temperature  p_inlet=0.101325 MPa  T_inlet=293.15 K  x_inlet=0  alpha_inlet=0  h_inlet=400 kJ/kg  u_inlet=400 kJ/kg  Cd=0.8  pressure_recovery=false  leakage_fraction=1e-9  smoothing_factor=0.01  B_lam=0.999  tau_x=0.1 s  area=return_pipe_inner_area m^2  vapor_valve_parameterization=fluids.two_phase_fluid.valves_orifices.enum.VaporOrificeParameterization.Cv  opening_characteristic=fluids.two_phase_fluid.valves_orifices.enum.OpeningCharacteristics.Linear  Cv_max=4  p_diff_Cv_TLU=0.2 : 0.2 : 1.2 MPa  p_gauge_Cv_TLU=0.2 : 0.2 : 1.2 MPa  Cv_TLU=[1e-06, .8, 1.6, 2.4, 3.2, 4]  xT_Cv=0.7  Kv_max=3.6  p_diff_Kv_TLU=0.2 : 0.2 : 1.2 MPa  p_gauge_Kv_TLU=0.2 : 0.2 : 1.2 MPa  Kv_TLU=[1e-06, .72, 1.44, 2.16, 2.88, 3.6]  xT_Kv=0.7  orifice_area_max=1e-4 m^2  p_diff_orifice_area_TLU=0.2 : 0.2 : 1.2 MPa  p_gauge_orifice_area_TLU=0.2 : 0.2 : 1.2 MPa  orifice_area_TLU=[1e-10, 2e-05, 4e-05, 6e-05, 8e-05, .0001] m^2
      settings: InternalSimscapePortConfiguration="{\"Bottom\":[],\"Left\":[{\"id\":\"A\",\"label\":\"A\",\"type\":\"foundation.two_phase_fluid.two_phase_fluid\"}],\"Right\":[{\"id\":\"B\",\"label\":\"B\",\"type\":\"foundation.two_phase_fluid.two_phase_fluid\"}],\"Top\":[]}"
  supply line hose : Subsystem
  mdot_ground_tank : Outport
  P_PUMP_GS : Outport  Port=2
  P_GH2_SUPPLY_GS : Outport  Port=3
  P_VALVE_RETURN_GS : Outport  Port=4
  T_BYPASS : Outport  Port=5
  Refuel_quality_check : Outport  Port=6
  AC_TK_LEVEL : Outport  Port=7
  P_TANK_AC : Outport  Port=8
  T_TANK_AC : Outport  Port=9
  P_BYPASS : Outport  Port=10
  P_COUPLING_AC : Outport  Port=11
  P_COUPLING_AC_RETURN : Outport  Port=12
  P_DIAGNOSTIC : Outport  Port=13  OutDataTypeStr=Bus: P_DIAGNOSTIC
  T_DIAGNOSTIC : Outport  Port=14  OutDataTypeStr=Bus: T_DIAGNOSTIC
  AC_TANK_SUPPLY_LINE_MDOT : Outport  Port=15
  LH2_SUPPLY_QDOT : Outport  Port=16
  GH2_SUPPLY_QDOT : Outport  Port=17
  GS_RETURN_QDOT : Outport  Port=18
  Engine_feed_mdot : Outport  Port=19
  AC_Tank_return_line_mdot : Outport  Port=20
  AC_Tank_Vent_mdot : Outport  Port=21
  Tank wall temp : Outport  Port=22
  GS_VALVE_FEEDBACK : Outport  Port=23  OutDataTypeStr=Bus: GS_VALVE_FEEDBACK
  AC_VALVE_FEEDBACK : Outport  Port=24  OutDataTypeStr=Bus: AC_VALVE_FEEDBACK
  wires:
  PS-Simulink Converter/1 -> [T_BYPASS]
  From/1 -> GS tank pressure controller/1(Target pressure)
  [Couplings_connected] -> GS_Return_Coupling/1
  Couplings_connected/1 -> [Couplings_connected]
  PS-Simulink Converter2/1 -> Goto1/1
  [mdot_ground_tank] -> mdot_ground_tank/1
  [Couplings_connected] -> AC_Supply_Coupling/1
  PS-Simulink Converter3/1 -> [AC_TK_LEVEL]
  PS-Simulink Converter4/1 -> [Refuel_quality_check]
  [Couplings_connected] -> AC_Return_Coupling/1
  [GS_Supply_SOV_CMD] -> GS_Supply_SOV/1
  [AC_Return_SOV_CMD] -> AC_Return_SOV/1(Valve_command)
  PS-Simulink Converter1/1 -> [mdot_ground_tank]
  [AC_Supply_SOV_CMD] -> AC_Supply_SOV/1
  [AC_Bypass_SOV_CMD] -> AC_Bypass_SOV/1
  From14/1 -> GS tank pressure controller/2(Tank pressure)
  [AC_Engine_SOV_CMD] -> AC_Engine_SOV/1(Valve_command)
  [GS_Return_SOV_CMD] -> GS_Return_SOV/1(Valve_command)
  [Couplings_connected] -> GS_Supply_Coupling/1
  GS_Supply_SOV_CMD/1 -> [GS_Supply_SOV_CMD]
  GS_Return_SOV_CMD/1 -> [GS_Return_SOV_CMD]
  AC_Supply_SOV_CMD/1 -> [AC_Supply_SOV_CMD]
  AC_Return_SOV_CMD/1 -> [AC_Return_SOV_CMD]
  AC_Bypass_SOV_CMD/1 -> [AC_Bypass_SOV_CMD]
  AC_Engine_SOV_CMD/1 -> [AC_Engine_SOV_CMD]
  [T_BYPASS] -> T_BYPASS/1
  [Refuel_quality_check] -> Refuel_quality_check/1
  [AC_TK_LEVEL] -> AC_TK_LEVEL/1
  PS-Simulink Converter5/1 -> [T_TANK_AC]
  PS-Simulink Converter6/1 -> [P_TANK_AC]
  [P_TANK_AC] -> P_TANK_AC/1
  [T_TANK_AC] -> T_TANK_AC/1
  PS-Simulink Converter8/1 -> [P_TANK_GS]
  PS-Simulink Converter7/1 -> [T_TANK_GS]
  PS-Simulink Converter9/1 -> [P_BYPASS]
  [P_BYPASS] -> P_BYPASS/1
  PS-Simulink Converter14/1 -> [T_VALVE_GS]
  PS-Simulink Converter15/1 -> [P_VALVE_GS]
  PS-Simulink Converter17/1 -> [P_HOSE_GS]
  PS-Simulink Converter16/1 -> [T_HOSE_GS]
  [P_TANK_GS] -> Bus Assignment/2
  Bus Assignment/1 -> P_DIAGNOSTIC/1
  [T_TANK_GS] -> Bus Assignment1/2
  Bus Assignment1/1 -> T_DIAGNOSTIC/1
  PS-Simulink Converter18/1 -> [T_COUPLINGS_GS]
  PS-Simulink Converter19/1 -> [P_COUPLINGS_GS]
  [GS_GH2_SOV_CMD] -> GS_GH2_SOV/1
  GS_GH2_SOV_CMD/1 -> [GS_GH2_SOV_CMD]
  Constant/1 -> Simulink-PS Converter1/1
  [P_VALVE_GS] -> Bus Assignment/5
  [P_HOSE_GS] -> Bus Assignment/6
  [P_COUPLINGS_GS] -> Bus Assignment/7
  [P_BYPASS] -> Bus Assignment/9
  [P_TANK_AC] -> Bus Assignment/10
  [T_VALVE_GS] -> Bus Assignment1/5
  [T_HOSE_GS] -> Bus Assignment1/6
  [T_COUPLINGS_GS] -> Bus Assignment1/7
  [T_BYPASS] -> Bus Assignment1/9
  [T_TANK_AC] -> Bus Assignment1/10
  Constant2/1 -> Simulink-PS Converter5/1
  PS-Simulink Converter13/1 -> [T_HOSE_RETURN_GS]
  PS-Simulink Converter20/1 -> [P_HOSE_RETURN_GS]
  PS-Simulink Converter22/1 -> [P_COUPLING_AC]
  PS-Simulink Converter21/1 -> [T_COUPLING_AC]
  [P_COUPLING_AC] -> Bus Assignment/8
  [T_COUPLING_AC] -> Bus Assignment1/8
  PS-Simulink Converter23/1 -> [T_COUPLING_AC_RETURN]
  PS-Simulink Converter24/1 -> [P_COUPLING_AC_RETURN]
  [P_COUPLING_AC_RETURN] -> Bus Assignment/12
  [T_COUPLING_AC_RETURN] -> Bus Assignment1/12
  [P_HOSE_RETURN_GS] -> Bus Assignment/13
  [T_HOSE_RETURN_GS] -> Bus Assignment1/13
  PS-Simulink Converter25/1 -> [LH2_SUPPLY_QDOT]
  PS-Simulink Converter26/1 -> [GH2_SUPPLY_QDOT]
  GH2_PROP_VALVE_CMD/1 -> [GH2_PROP_VALVE_CMD]
  Bus Creator/1 -> Bus Assignment/1
  Bus Creator1/1 -> Bus Assignment1/1
  PS-Simulink Converter10/1 -> [AC_TANK_SUPPLY_LINE_MDOT]
  [AC_TANK_SUPPLY_LINE_MDOT] -> AC_TANK_SUPPLY_LINE_MDOT/1
  [LH2_SUPPLY_QDOT] -> LH2_SUPPLY_QDOT/1
  [GH2_SUPPLY_QDOT] -> GH2_SUPPLY_QDOT/1
  Constant6/1 -> Simulink-PS Converter/1
  PS-Simulink Converter11/1 -> [Engine_feed_mdot], Display/1
  Constant1/1 -> Simulink-PS Converter3/1
  PS-Simulink Converter12/1 -> [T_VALVE_RETURN_GS]
  PS-Simulink Converter27/1 -> [P_VALVE_RETURN_GS]
  [P_VALVE_RETURN_GS] -> Bus Assignment/14
  [T_VALVE_RETURN_GS] -> Bus Assignment1/14
  [VENT_PROP_VALVE_CMD] -> Return gas proportional valve/1
  Constant5/1 -> Simulink-PS Converter2/1
  [GH2_PROP_VALVE_CMD] -> GH2 Proportional valve/1
  PS-Simulink Converter28/1 -> [GS_RETURN_QDOT]
  [GS_RETURN_QDOT] -> GS_RETURN_QDOT/1
  PS-Simulink Converter29/1 -> Display1/1
  PS-Simulink Converter30/1 -> [T_PUMP_GS]
  PS-Simulink Converter31/1 -> [P_PUMP_GS]
  [P_PUMP_GS] -> Bus Assignment/3
  [T_PUMP_GS] -> Bus Assignment1/3
  PS-Simulink Converter32/1 -> Display2/1
  Constant4/1 -> Simulink-PS Converter4/1
  [Engine_feed_mdot] -> Engine_feed_mdot/1
  PS-Simulink Converter34/1 -> [P_ENGINE_FEED]
  PS-Simulink Converter33/1 -> [T_ENGINE_FEED]
  [T_ENGINE_FEED] -> Bus Assignment1/11
  [P_ENGINE_FEED] -> Bus Assignment/11
  PS-Simulink Converter36/1 -> [P_GH2_SUPPLY_GS]
  PS-Simulink Converter35/1 -> [T_GH2_SUPPLY_GS]
  [P_GH2_SUPPLY_GS] -> Bus Assignment/4
  [T_GH2_SUPPLY_GS] -> Bus Assignment1/4
  PS-Simulink Converter37/1 -> [AC_Tank_Vent_mdot], Display3/1
  PS-Simulink Converter38/1 -> [AC_Tank_return_line_mdot], Display4/1
  [AC_Tank_return_line_mdot] -> AC_Tank_return_line_mdot/1
  [AC_Tank_Vent_mdot] -> AC_Tank_Vent_mdot/1
  VENT_PROP_VALVE_CMD/1 -> [VENT_PROP_VALVE_CMD]
  [TANK_WALL_TEMP] -> Tank wall temp/1
  AC tank/1(Tank wall temp) -> [TANK_WALL_TEMP]
  LH2 Proportional valve/1 -> [LH2_PROP_VALVE_POS]
  GH2 Proportional valve/1 -> [GH2_PROP_VALVE_POS]
  GS_Supply_SOV/1 -> [GS_Supply_SOV_POS]
  GS_GH2_SOV/1 -> [GS_GH2_SOV_POS]
  AC_Supply_SOV/1 -> [AC_Supply_SOV_POS]
  AC_Engine_SOV/1(VALVE_POS) -> [AC_Engine_SOV_POS]
  AC_Return_SOV/1(VALVE_POS) -> [AC_Return_SOV_POS]
  GS_Return_SOV/1(VALVE_POS) -> [GS_Return_SOV_POS]
  Return gas proportional valve/1 -> [GS_RETURN_PROP_POS]
  Bus Creator2/1 -> Bus Assignment2/1
  Bus Assignment2/1 -> GS_VALVE_FEEDBACK/1
  AC_Bypass_SOV/1 -> [AC_Bypass_SOV_POS]
  Bus Assignment3/1 -> AC_VALVE_FEEDBACK/1
  Bus Creator3/1 -> Bus Assignment3/1
  [AC_Return_SOV_POS] -> Bus Assignment3/2
  [AC_Supply_SOV_POS] -> Bus Assignment3/3
  [AC_Bypass_SOV_POS] -> Bus Assignment3/4
  [AC_Engine_SOV_POS] -> Bus Assignment3/5
  [LH2_PROP_VALVE_POS] -> Bus Assignment2/2
  [GH2_PROP_VALVE_POS] -> Bus Assignment2/3
  [GS_Supply_SOV_POS] -> Bus Assignment2/4
  [GS_GH2_SOV_POS] -> Bus Assignment2/5
  [GS_Return_SOV_POS] -> Bus Assignment2/6
  [GS_RETURN_PROP_POS] -> Bus Assignment2/7
  [LH2_PROP_VALVE_CMD] -> LH2 Proportional valve/1
  LH2_PROP_VALVE_CMD/1 -> [LH2_PROP_VALVE_CMD]
  [P_COUPLING_AC] -> P_COUPLING_AC/1
  [P_COUPLING_AC_RETURN] -> P_COUPLING_AC_RETURN/1
  [P_PUMP_GS] -> P_PUMP_GS/1
  [P_VALVE_RETURN_GS] -> P_VALVE_RETURN_GS/1
  [P_GH2_SUPPLY_GS] -> P_GH2_SUPPLY_GS/1
  connections:
  AC return line pipe/RConn1 -- AC bypass pipe/LConn1 -- AC_Return_SOV/LConn1
  Vapor Quality Sensor (2P)/LConn1 -- Flow Rate Sensor (2P)2/LConn1 -- AC_Supply_SOV/RConn1 -- "Pressure, Temperature & Internal Energy Sensor (2P)1"/LConn1
  "Pressure, Temperature & Internal Energy Sensor (2P)"/LConn1 -- AC_Bypass_SOV/LConn1 -- AC_Supply_SOV/LConn1 -- AC supply line pipe/RConn1
  Safety valve/RConn1 -- Atmosphere/LConn1
  PS-Simulink Converter1/LConn1 -- Flow rate sensor/RConn2
  GS_Supply_Coupling/LConn1 -- "Pressure, Temperature & Internal Energy Sensor (2P)6"/LConn1 -- AC bypass check valve/LConn1 -- supply line hose/RConn1
  AC tank safety valve/RConn1 -- Atmosphere2/LConn1
  PS-Simulink Converter4/LConn1 -- Vapor Quality Sensor (2P)/RConn1
  AC_Return_Coupling/LConn1 -- GS_Return_Coupling/RConn1
  GS_Return_SOV/RConn1 -- Return line hose/LConn1 -- "Pressure, Temperature & Internal Energy Sensor (2P)4"/LConn1
  Return line hose/RConn1 -- AC bypass check valve/RConn1 -- GS_Return_Coupling/LConn1
  AC_Return_SOV/RConn1 -- Flow Rate Sensor (2P)6/RConn1
  PS-Simulink Converter/LConn1 -- "Pressure, Temperature & Internal Energy Sensor (2P)"/RConn2
  "Pressure, Temperature & Internal Energy Sensor (2P)9"/LConn1 -- AC_Return_Coupling/RConn1 -- AC return line pipe/LConn1
  Safety valve/LConn1 -- Ground station tank/LConn1
  PS-Simulink Converter3/LConn1 -- AC tank/RConn3
  AC supply line pipe/LConn1 -- "Pressure, Temperature & Internal Energy Sensor (2P)8"/LConn1 -- AC_Supply_Coupling/RConn1
  "Pressure, Temperature & Internal Energy Sensor (2P)7"/LConn1 -- AC_Supply_Coupling/LConn1 -- GS_Supply_Coupling/RConn1
  PS-Simulink Converter2/LConn1 -- Ground station tank/RConn3
  PS-Simulink Converter5/LConn1 -- "Pressure, Temperature & Internal Energy Sensor (2P)1"/RConn2
  PS-Simulink Converter6/LConn1 -- "Pressure, Temperature & Internal Energy Sensor (2P)1"/RConn1
  PS-Simulink Converter7/LConn1 -- "Pressure, Temperature & Internal Energy Sensor (2P)2"/RConn2
  PS-Simulink Converter8/LConn1 -- "Pressure, Temperature & Internal Energy Sensor (2P)2"/RConn1
  PS-Simulink Converter9/LConn1 -- "Pressure, Temperature & Internal Energy Sensor (2P)"/RConn1
  PS-Simulink Converter15/LConn1 -- "Pressure, Temperature & Internal Energy Sensor (2P)5"/RConn1
  PS-Simulink Converter14/LConn1 -- "Pressure, Temperature & Internal Energy Sensor (2P)5"/RConn2
  PS-Simulink Converter17/LConn1 -- "Pressure, Temperature & Internal Energy Sensor (2P)6"/RConn1
  PS-Simulink Converter16/LConn1 -- "Pressure, Temperature & Internal Energy Sensor (2P)6"/RConn2
  PS-Simulink Converter19/LConn1 -- "Pressure, Temperature & Internal Energy Sensor (2P)7"/RConn1
  PS-Simulink Converter18/LConn1 -- "Pressure, Temperature & Internal Energy Sensor (2P)7"/RConn2
  "Pressure, Temperature & Internal Energy Sensor (2P)12"/LConn1 -- GS_GH2_SOV/LConn1 -- GH2 Proportional valve/LConn2
  Simulink-PS Converter/RConn1 -- GH2 source/RConn2
  Simulink-PS Converter1/RConn1 -- GH2 source/RConn1
  Simulink-PS Converter5/RConn1 -- GH2 vent/RConn1
  PS-Simulink Converter20/LConn1 -- "Pressure, Temperature & Internal Energy Sensor (2P)4"/RConn1
  PS-Simulink Converter13/LConn1 -- "Pressure, Temperature & Internal Energy Sensor (2P)4"/RConn2
  PS-Simulink Converter22/LConn1 -- "Pressure, Temperature & Internal Energy Sensor (2P)8"/RConn1
  PS-Simulink Converter21/LConn1 -- "Pressure, Temperature & Internal Energy Sensor (2P)8"/RConn2
  PS-Simulink Converter24/LConn1 -- "Pressure, Temperature & Internal Energy Sensor (2P)9"/RConn1
  PS-Simulink Converter23/LConn1 -- "Pressure, Temperature & Internal Energy Sensor (2P)9"/RConn2
  Flow Rate Sensor (2P)1/RConn1 -- LH2 supply check valve/LConn1
  GS_GH2_SOV/RConn1 -- Flow Rate Sensor (2P)/LConn1
  GS_Supply_SOV/RConn1 -- Flow Rate Sensor (2P)1/LConn1
  PS-Simulink Converter25/LConn1 -- Flow Rate Sensor (2P)1/RConn2
  Flow Rate Sensor (2P)/RConn2 -- PS-Simulink Converter26/LConn1
  PS-Simulink Converter10/LConn1 -- Flow Rate Sensor (2P)2/RConn2
  Flow Rate Sensor (2P)2/RConn1 -- AC tank/LConn2
  "Pressure, Temperature & Internal Energy Sensor (2P)5"/LConn1 -- GH2 supply check valve/RConn1 -- supply line hose/LConn1 -- GS supply line pipe/RConn1
  Flow Rate Sensor (2P)/RConn1 -- GH2 supply check valve/LConn1
  GH2 vent/RConn2 -- Simulink-PS Converter2/RConn1
  PS-Simulink Converter11/LConn1 -- Flow Rate Sensor (2P)3/RConn2
  AC_Engine_SOV/RConn1 -- Flow Rate Sensor (2P)3/LConn1
  AC engine_feed_pipe/RConn1 -- Atmosphere3/LConn1
  GH2 vent/LConn1 -- Vent check valve/RConn1
  Simulink-PS Converter3/RConn1 -- LH2 source/RConn1
  LH2 source/RConn2 -- Simulink-PS Converter4/RConn1
  AC_Bypass_SOV/RConn1 -- AC bypass pipe/RConn1
  Solver Configuration2/RConn1 -- Flow rate sensor/LConn1 -- Ground station tank/RConn2 -- LH2 source/LConn1 -- Ground station tank/LConn2 -- H2 2 phase/RConn1
  PS-Simulink Converter12/LConn1 -- "Pressure, Temperature & Internal Energy Sensor (2P)3"/RConn2
  PS-Simulink Converter27/LConn1 -- "Pressure, Temperature & Internal Energy Sensor (2P)3"/RConn1
  Vent check valve/LConn1 -- Flow Rate Sensor (2P)4/RConn1
  "Pressure, Temperature & Internal Energy Sensor (2P)2"/LConn1 -- Vapor Quality Sensor (2P)1/LConn1 -- LH2 Proportional valve/LConn1 -- Flow rate sensor/RConn1
  Return gas proportional valve/LConn1 -- "Pressure, Temperature & Internal Energy Sensor (2P)3"/LConn1 -- GS_Return_SOV/LConn1
  GH2 Proportional valve/LConn1 -- GH2 source/LConn1
  PS-Simulink Converter28/LConn1 -- Flow Rate Sensor (2P)4/RConn2
  Flow Rate Sensor (2P)4/LConn1 -- Return gas proportional valve/LConn2
  PS-Simulink Converter29/LConn1 -- Vapor Quality Sensor (2P)1/RConn1
  PS-Simulink Converter30/LConn1 -- "Pressure, Temperature & Internal Energy Sensor (2P)10"/RConn2
  PS-Simulink Converter31/LConn1 -- "Pressure, Temperature & Internal Energy Sensor (2P)10"/RConn1
  PS-Simulink Converter32/LConn1 -- Vapor Quality Sensor (2P)2/RConn1
  LH2 supply check valve/RConn1 -- GS supply line pipe/LConn1
  Vapor Quality Sensor (2P)2/LConn1 -- "Pressure, Temperature & Internal Energy Sensor (2P)10"/LConn1 -- GS_Supply_SOV/LConn1 -- LH2 Proportional valve/LConn2
  AC_Engine_SOV/LConn1 -- AC tank/RConn2
  PS-Simulink Converter34/LConn1 -- "Pressure, Temperature & Internal Energy Sensor (2P)11"/RConn1
  PS-Simulink Converter33/LConn1 -- "Pressure, Temperature & Internal Energy Sensor (2P)11"/RConn2
  Flow Rate Sensor (2P)3/RConn1 -- AC engine_feed_pipe/LConn1 -- "Pressure, Temperature & Internal Energy Sensor (2P)11"/LConn1
  PS-Simulink Converter35/LConn1 -- "Pressure, Temperature & Internal Energy Sensor (2P)12"/RConn2
  PS-Simulink Converter36/LConn1 -- "Pressure, Temperature & Internal Energy Sensor (2P)12"/RConn1
  AC tank/RConn1 -- Flow Rate Sensor (2P)5/LConn1
  Flow Rate Sensor (2P)5/RConn1 -- AC tank safety valve/LConn1
  PS-Simulink Converter37/LConn1 -- Flow Rate Sensor (2P)5/RConn2
  PS-Simulink Converter38/LConn1 -- Flow Rate Sensor (2P)6/RConn2
  Flow Rate Sensor (2P)6/LConn1 -- AC tank/LConn1
